simulink library "pmm"  (R2021b)
settings: Solver=VariableStepAuto  StartTime=0.0  StopTime=10.0  RelTol=1e-3
undefined symbols (not defined in the file or in its folder): APMM_CoolgFanActCurr_X_pct, APMM_EWP1Curr_X_c, APMM_EWP3Curr_X_c, APMM_LVBattChktime_X_enum, APMM_LVBattChrgtime_X_enum, APMM_LVChrgLv_X_mV, ENUM_ANTITHEFT_ALARM, ENUM_ANTITHEFT_ARM, ENUM_ANTITHEFT_DISARM, ENUM_ANTITHEFT_WAIT, ENUM_CHRGPLUGSTA_NONE, ENUM_CRASHSTATE_NOCRASH, ENUM_DCDCFAULTSTA_ANYFAULTLV1, ENUM_DCDCFAULTSTA_ANYFAULTLV2, ENUM_DRIVETRAIN_AWD, ENUM_DRIVETRAIN_FWD, ENUM_DRIVETRAIN_RWD, ENUM_GEARACTUALPOSN_D, ENUM_GEARACTUALPOSN_N, ENUM_GEARACTUALPOSN_R, ENUM_HVBATTREADYPRE_READY, ENUM_OTACHKSTA_NOREQUEST, ENUM_OTACHKSTA_NOTIMEOUT, ENUM_OTACHKSTA_TIMEOUT, ENUM_PDKEYRAWLULOCK_INLOCK, ENUM_PDKEYRAWLULOCK_INUNLOCK, ENUM_PDKEYRAWPS_INPS, ENUM_PDKEYSTA_LOCK, ENUM_PDKEYSTA_PS, ENUM_PDKEYSTA_UNAVALIABLE, ENUM_PDKEYSTA_UNLOCK, ENUM_POWERSTA_OFF, ENUM_POWERSTA_OFFC, ENUM_POWERSTA_STANDBY, ENUM_PWRREQOTA_REQPOWEROFF, ENUM_PWRREQOTA_REQPOWERSTDBY, ENUM_PWRSTASW_READY, FALSE, KPMM_AllDoorClosedHoldTime_s, KPMM_APSAllowThd_pct, KPMM_BattDownFailtime_s, KPMM_BattUpFailtime_s, KPMM_BattUpResetRty_cnt, KPMM_BattUpResetSW_flg, KPMM_BattUpResetTO_s, KPMM_BattUpRstDlyTO_s, KPMM_BrakeSWHoldTime_s, KPMM_ChrgPlugHoldTime_s, KPMM_DCDCDisableFailtime_s, KPMM_DCDCEnableFailtime_s, KPMM_DCDCVSET_V, KPMM_DCDCVSETLVChrg_V, KPMM_DoorSWHoldTime_s, KPMM_DriverSafetyChkFailtime_s, KPMM_DrivetrainSelect_enum_ovrdflg, KPMM_DrivetrainSelect_enum_ovrdval, KPMM_FDADC12VDetAccu_s, KPMM_FDADC12VDetAccuIntval_s, KPMM_FirstLVCheckHoldT_s, KPMM_FrMCUDischrgVolt_V ... (+54)
libraries: simulink x28, hcu_lib x13
(part 1 of 5)
settings Model: Creator=13615  LastModifiedBy=FVT23010
settings SolverCC: AlgebraicLoopSolver=TrustRegion
settings DataIOCC: SaveFormat=Array  SignalLoggingSaveFormat=ModelDataLogs  ReturnWorkspaceOutputs=off
settings OptimizationCC: BlockReduction=off  BooleanDataType=off
settings DebuggingCC: SaveWithParameterizedLinksMsg=none  UnderspecifiedInitializationDetection=Classic  MergeDetectMultiDrivingBlocksExec=none  SignalResolutionControl=TryResolveAllWithWarning  SFMachineParentedDataDiag=warning  ArithmeticOperatorsInVariantConditions=warning
settings HardwareCC: TargetUnknown=on
settings ModelReferenceCC: PropagateSignalLabelsOutOfModel=off
settings SFSimCC: SimUseLocalCustomCode=off  CustomCodeUndefinedFunction=UseInterfaceOnly
settings RTWCC: RTWUseLocalCustomCode=off
settings ConfigComp: CovMetricSettings=dw  CovSaveCumulativeToWorkspaceVar=on  CovSaveSingleToWorkspaceVar=on

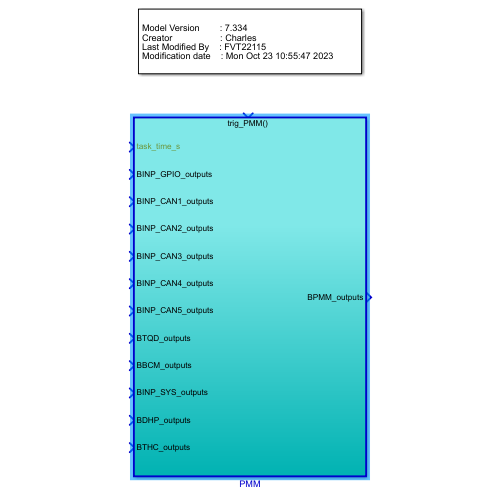
[thumbnail: Simulink's stored preview of the top-level diagram]
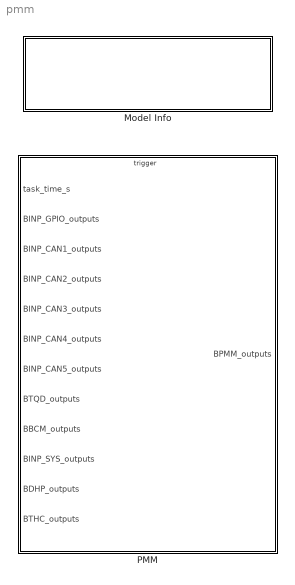
== system pmm ==
  Model Info : Subsystem  LoadFcn=slcm LoadBlock;  InitFcn=slcm('UpdateAllCMBlocksInThisModelInit')  mask(CMBlock){InitialSaveTempField=, InitialBlockCM=None, BlockCM=None, Frame=on, SaveTempField=, DisplayStringWithTags=|, MaskDisplayString=Model Version        : 7.543\nCreator                   : Charles\nLast Modified By    : FVT23010\nModification date    : Mon Jun 24 15:30:34 2024, HorizontalTextAlignment=Left, LeftAlignmentValue=0.02, SourceBlockDiagram=pmm, TagMaxNumber=20, CMTag1=, CMTag2=, CMTag3=, CMTag4=, CMTag5=, CMTag6=, CMTag7=, CMTag8=, CMTag9=, CMTag10=, CMTag11=, CMTag12=, CMTag13=, CMTag14=, CMTag15=, CMTag16=, CMTag17=, CMTag18=, CMTag19=, CMTag20=}
      mask DisplayStringWithTags=|
      | Model Version        : %<ModelVersion>
      | Creator                   : Charles
      | Last Modified By    : %<LastModifiedBy>
      | Modification date    : %<LastModificationDate>
      mask help: This block allows revision control information to be displayed within the model.
      settings: CopyFcn=slcm CopyBlock;  DeleteFcn=slcm Cancel;  PostSaveFcn=slcm('UpdateAllCMBlocksInThisModel')  NameChangeFcn=slcm Rename;  OpenFcn=slcm
      mask Display: text(str2num(LeftAlignmentValue), 0.5, MaskDisplayString, 'HorizontalAlignment', HorizontalTextAlignment)
  PMM : Subsystem  TreatAsAtomicUnit=on
      settings: RTWSystemCode=Nonreusable function  RTWFcnNameOpts=Use subsystem name  RTWFileNameOpts=Use subsystem name

== system pmm/Model Info ==
  EmptySubsystem : Subsystem

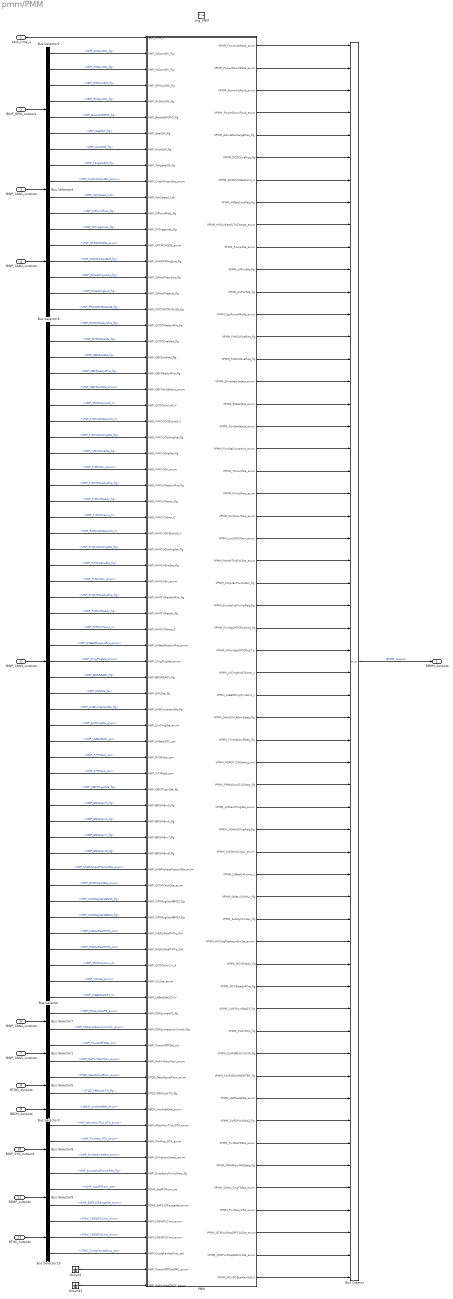
== system pmm/PMM ==
  task_time_s : Inport
  BINP_GPIO_outputs : Inport  Port=2  OutDataTypeStr=Bus: BINP_GPIO_outputs
  BINP_CAN1_outputs : Inport  Port=3  OutDataTypeStr=Bus: BINP_CAN1_outputs
  BINP_CAN2_outputs : Inport  Port=4  OutDataTypeStr=Bus: BINP_CAN2_outputs
  BINP_CAN3_outputs : Inport  Port=5  OutDataTypeStr=Bus: BINP_CAN3_outputs
  BINP_CAN4_outputs : Inport  Port=6  OutDataTypeStr=Bus: BINP_CAN4_outputs
  BINP_CAN5_outputs : Inport  Port=7  OutDataTypeStr=Bus: BINP_CAN5_outputs
  BTQD_outputs : Inport  Port=8  OutDataTypeStr=Bus: BTQD_outputs
  BBCM_outputs : Inport  Port=9  OutDataTypeStr=Bus: BBCM_outputs
  BINP_SYS_outputs : Inport  Port=10  OutDataTypeStr=Bus: BINP_SYS_outputs
  BDHP_outputs : Inport  Port=11  OutDataTypeStr=Bus: BDHP_outputs
  BTHC_outputs : Inport  Port=12  OutDataTypeStr=Bus: BTHC_outputs
  trig_PMM : TriggerPort  TriggerType=function-call  VariantControl=(inherit)
  Bus Creator : BusCreator  Inputs=56  OutDataTypeStr=Bus: BPMM_outputs  NonVirtualBus=on
  Bus Selector : BusSelector  OutputSignals=VINP_DCDCReady4Pre_flg,VINP_DCDCEnaSta_flg,VINP_OBCEnaSta_flg,VINP_OBCReady4Pre_flg,VINP_OBCFaultSta_enum,VINP_DCDCAuxVolt_V,VINP_FrMCUDCBusVolt_V,VINP_FrMCUDischrgSta_flg,VINP_FrMCUEnaSta_flg,VINP_FrMCUErr_enum,VINP_FrMCUReady4Pre_flg,VINP_FrMCUReady_flg,VINP_FrMCUTemp_C,VINP_RrMCUDCBusVolt_V,VINP_RrMCUDischrgSta_flg,VINP_RrMCUEnaSta_flg,VINP_RrMCUErr_enum,VINP_RrMCUReady4Pre_flg,VINP_RrMCUReady_flg,VINP_RrMCUTemp_C,VINP_HVBattReady4Pre_enum,VINP_ChrgPlugSta_enum,VINP_BMSREADY_flg,VINP_HVILSta_flg,VINP_HVBContactorSta_flg,VINP_ExtChrgSta_enum,VINP_HVBattSOC_pct,VINP_RrTMSpd_rpm,VINP_FrTMSpd_rpm,VINP_OBCPluginSta_flg,VINP_BMSWarn5_flg,VINP_BMSWarn6_flg,VINP_BMSWarn7_flg,VINP_BMSWarn8_flg,VINP_HVBPreheatPrecoolSta_enum,VINP_DCDCFaultSta_enum,VINP_CANMsgValidBMS5_flg,VINP_CANMsgValidBMS3_flg,VINP_FrEDURealTMTq_Nm,VINP_RrEDURealTMTq_Nm,VINP_DCDCAuxCur_A,VINP_V2LSta_enum,VINP_LVBattDet12V_V
  Bus Selector1 : BusSelector  OutputSignals=VINP_PowerOffTSet_cnt,VINP_RePwrReqTbox_enum
  Bus Selector10 : BusSelector  OutputSignals=VTHC_FDEWP1Cmd_enum,VTHC_FDEWP3Cmd_enum,VTHC_CoolgFanActDuty_pct
  Bus Selector2 : BusSelector  OutputSignals=VINP_DrDoorSW_flg,VINP_PsDoorSW_flg,VINP_RRDoorSW_flg,VINP_RLDoorSW_flg,VINP_BrakeSWGPIO_flg,VINP_SeatSW_flg,VINP_HoodSW_flg,VINP_TailgateSW_flg
  Bus Selector3 : BusSelector  OutputSignals=VBCM_AntitheftSta_enum
  Bus Selector4 : BusSelector  OutputSignals=VINP_CrashOutputSts_enum,VINP_VehSpeed_kph
  Bus Selector5 : BusSelector  OutputSignals=VTQD_GearActualPosn_enum,VTQD_PBWLockTO_flg
  Bus Selector6 : BusSelector  OutputSignals=VINP_IVIPwroffreq_flg,VINP_IVITriggerreq_flg,VINP_OFFACMODE_enum,VINP_AVMOFFRecButt_flg,VINP_SchedChgwake_flg,VINP_SchedChgbutt_flg,VINP_PWCONTINUEUSE_flg
  Bus Selector7 : BusSelector  OutputSignals=VINP_PDKeyAreaPS_enum,VINP_PDKeyAreaLockUnlock_enum
  Bus Selector8 : BusSelector  OutputSignals=VINP_AllowMovThd_OTA_enum,VINP_PwrReq_OTA_enum,VINP_DrivetrainSelect_enum,VINP_EvccAplusPwrUpReq_flg
  Bus Selector9 : BusSelector  OutputSignals=VDHP_ActAPSPosn_pct,VDHP_EAPS12RangeSta_enum
  Ground : Ground
  Ground3 : Ground
  PMM : Subsystem
  BPMM_outputs : Outport  OutDataTypeStr=Bus: BPMM_outputs  VectorParamsAs1DForOutWhenUnconnected=off
  wires:
  BINP_CAN3_outputs/1 -> Bus Selector/1
  Bus Creator/1 -> BPMM_outputs/1  "BPMM_outputs"
  task_time_s/1 -> PMM/1(task_time_s)
  BINP_GPIO_outputs/1 -> Bus Selector2/1
  BBCM_outputs/1 -> Bus Selector3/1
  BTQD_outputs/1 -> Bus Selector5/1
  Bus Selector2/4 -> PMM/5(VINP_RLDoorSW_flg)  "<VINP_RLDoorSW_flg>"
  Bus Selector2/5 -> PMM/6(VINP_BrakeSWGPIO_flg)  "<VINP_BrakeSWGPIO_flg>"
  Bus Selector2/3 -> PMM/4(VINP_RRDoorSW_flg)  "<VINP_RRDoorSW_flg>"
  Bus Selector2/2 -> PMM/3(VINP_PsDoorSW_flg)  "<VINP_PsDoorSW_flg>"
  Bus Selector2/1 -> PMM/2(VINP_DrDoorSW_flg)  "<VINP_DrDoorSW_flg>"
  Bus Selector/1 -> PMM/19(VINP_DCDCReady4Pre_flg)  "<VINP_DCDCReady4Pre_flg>"
  Bus Selector/2 -> PMM/20(VINP_DCDCEnabled_flg)  "<VINP_DCDCEnaSta_flg>"
  Bus Selector/3 -> PMM/21(VINP_OBCEnabled_flg)  "<VINP_OBCEnaSta_flg>"
  Bus Selector/4 -> PMM/22(VINP_OBCReady4Pre_flg)  "<VINP_OBCReady4Pre_flg>"
  Bus Selector/5 -> PMM/23(VINP_OBCFaultStatus_enum)  "<VINP_OBCFaultSta_enum>"
  Bus Selector/6 -> PMM/24(VINP_DCDCAuxVolt_V)  "<VINP_DCDCAuxVolt_V>"
  Bus Selector/7 -> PMM/25(VINP_FrMCUDCBusVolt_V)  "<VINP_FrMCUDCBusVolt_V>"
  Bus Selector/8 -> PMM/26(VINP_FrMCUDischrgSta_flg)  "<VINP_FrMCUDischrgSta_flg>"
  Bus Selector/9 -> PMM/27(VINP_FrMCUEnaSta_flg)  "<VINP_FrMCUEnaSta_flg>"
  Bus Selector/10 -> PMM/28(VINP_FrMCUErr_enum)  "<VINP_FrMCUErr_enum>"
  Bus Selector/11 -> PMM/29(VINP_FrMCUReady4Pre_flg)  "<VINP_FrMCUReady4Pre_flg>"
  Bus Selector/12 -> PMM/30(VINP_FrMCUReady_flg)  "<VINP_FrMCUReady_flg>"
  Bus Selector/13 -> PMM/31(VINP_FrMCUTemp_C)  "<VINP_FrMCUTemp_C>"
  Bus Selector/14 -> PMM/32(VINP_RrMCUDCBusVolt_V)  "<VINP_RrMCUDCBusVolt_V>"
  Bus Selector/15 -> PMM/33(VINP_RrMCUDischrgSta_flg)  "<VINP_RrMCUDischrgSta_flg>"
  Bus Selector/16 -> PMM/34(VINP_RrMCUEnaSta_flg)  "<VINP_RrMCUEnaSta_flg>"
  Bus Selector/17 -> PMM/35(VINP_RrMCUErr_enum)  "<VINP_RrMCUErr_enum>"
  Bus Selector/18 -> PMM/36(VINP_RrMCUReady4Pre_flg)  "<VINP_RrMCUReady4Pre_flg>"
  Bus Selector/19 -> PMM/37(VINP_RrMCUReady_flg)  "<VINP_RrMCUReady_flg>"
  Bus Selector/20 -> PMM/38(VINP_RrMCUTemp_C)  "<VINP_RrMCUTemp_C>"
  Bus Selector/21 -> PMM/39(VINP_HVBattReady4Pre_enum)  "<VINP_HVBattReady4Pre_enum>"
  Bus Selector/22 -> PMM/40(VINP_ChrgPlugSta_enum)  "<VINP_ChrgPlugSta_enum>"
  Bus Selector/23 -> PMM/41(VINP_BMSREADY_flg)  "<VINP_BMSREADY_flg>"
  Bus Selector/24 -> PMM/42(VINP_HVILSta_flg)  "<VINP_HVILSta_flg>"
  Bus Selector/26 -> PMM/44(VINP_ExtChrgSta_enum)  "<VINP_ExtChrgSta_enum>"
  BINP_CAN1_outputs/1 -> Bus Selector4/1
  Bus Selector4/1 -> PMM/10(VINP_CrashOutputSts_enum)  "<VINP_CrashOutputSts_enum>"
  Bus Selector2/6 -> PMM/7(VINP_SeatSW_flg)  "<VINP_SeatSW_flg>"
  Bus Selector/27 -> PMM/45(VINP_HVBattSOC_pct)  "<VINP_HVBattSOC_pct>"
  Bus Selector/25 -> PMM/43(VINP_HVBContactorSta_flg)  "<VINP_HVBContactorSta_flg>"
  BINP_CAN2_outputs/1 -> Bus Selector6/1
  Bus Selector6/1 -> PMM/12(VINP_IVIPwroffreq_flg)  "<VINP_IVIPwroffreq_flg>"
  Bus Selector6/2 -> PMM/13(VINP_IVITriggerreq_flg)  "<VINP_IVITriggerreq_flg>"
  Bus Selector7/1 -> PMM/62(VINP_PDKeyAreaPS_flg)  "<VINP_PDKeyAreaPS_enum>"
  Bus Selector7/2 -> PMM/63(VINP_PDKeyAreaLockUnlock_flg)  "<VINP_PDKeyAreaLockUnlock_enum>"
  BINP_CAN4_outputs/1 -> Bus Selector7/1
  Bus Selector/28 -> PMM/46(VINP_RrTMSpd_rpm)  "<VINP_RrTMSpd_rpm>"
  Bus Selector4/2 -> PMM/11(VINP_VehSpeed_kph)  "<VINP_VehSpeed_kph>"
  Bus Selector/29 -> PMM/47(VINP_FrTMSpd_rpm)  "<VINP_FrTMSpd_rpm>"
  Bus Selector6/3 -> PMM/14(VINP_OFFACMODE_enum)  "<VINP_OFFACMODE_enum>"
  Bus Selector/30 -> PMM/48(VINP_OBCPluginSta_flg)  "<VINP_OBCPluginSta_flg>"
  Bus Selector/31 -> PMM/49(VINP_BMSWarn5_flg)  "<VINP_BMSWarn5_flg>"
  Bus Selector/32 -> PMM/50(VINP_BMSWarn6_flg)  "<VINP_BMSWarn6_flg>"
  Bus Selector/33 -> PMM/51(VINP_BMSWarn7_flg)  "<VINP_BMSWarn7_flg>"
  Bus Selector/34 -> PMM/52(VINP_BMSWarn8_flg)  "<VINP_BMSWarn8_flg>"
  BINP_CAN5_outputs/1 -> Bus Selector1/1
  Bus Selector/35 -> PMM/53(VINP_HVBPreheatPrecoolSta_enum)  "<VINP_HVBPreheatPrecoolSta_enum>"
  Bus Selector6/4 -> PMM/15(VINP_AVMOFFRecButt_flg)  "<VINP_AVMOFFRecButt_flg>"
  Bus Selector6/5 -> PMM/16(VINP_SchedChgwake_flg)  "<VINP_SchedChgwake_flg>"
  Bus Selector2/7 -> PMM/8(VINP_HoodSW_flg)  "<VINP_HoodSW_flg>"
  Bus Selector2/8 -> PMM/9(VINP_TailgateSW_flg)  "<VINP_TailgateSW_flg>"
  Bus Selector6/6 -> PMM/17(VINP_SchedChgbutt_flg)  "<VINP_SchedChgbutt_flg>"
  Bus Selector/38 -> PMM/56(VINP_CANMsgValidBMS3_flg)  "<VINP_CANMsgValidBMS3_flg>"
  BINP_SYS_outputs/1 -> Bus Selector8/1
  Bus Selector8/1 -> PMM/69(VINP_AllowMovThd_OTA_enum)  "<VINP_AllowMovThd_OTA_enum>"
  Bus Selector8/2 -> PMM/70(VINP_PwrReq_OTA_enum)  "<VINP_PwrReq_OTA_enum>"
  Bus Selector3/1 -> PMM/68(VBCM_AntitheftSta_enum)  "<VBCM_AntitheftSta_enum>"
  Bus Selector5/1 -> PMM/66(VTQD_GearActualPosn_enum)  "<VTQD_GearActualPosn_enum>"
  Bus Selector5/2 -> PMM/67(VTQD_PBWLockTO_flg)  "<VTQD_PBWLockTO_flg>"
  Ground3/1 -> PMM/79(VINP_RePwrReqDKCT_enum)
  Ground/1 -> PMM/78(VINP_PowerOffTSetDKC_enum)
  Bus Selector1/1 -> PMM/64(VINP_PowerOffTSet_cnt)  "<VINP_PowerOffTSet_cnt>"
  Bus Selector1/2 -> PMM/65(VINP_RePwrReqTbox_enum)  "<VINP_RePwrReqTbox_enum>"
  Bus Selector8/3 -> PMM/71(VINP_DrivetrainSelect_enum)  "<VINP_DrivetrainSelect_enum>"
  Bus Selector8/4 -> PMM/72(VINP_EvccAplusPwrUpReq_flg)  "<VINP_EvccAplusPwrUpReq_flg>"
  BDHP_outputs/1 -> Bus Selector9/1
  Bus Selector9/1 -> PMM/73(VDHP_ActAPSPosn_pct)  "<VDHP_ActAPSPosn_pct>"
  Bus Selector/36 -> PMM/54(VINP_DCDCFaultSta_enum)  "<VINP_DCDCFaultSta_enum>"
  Bus Selector/39 -> PMM/57(VINP_FrEDURealTMTq_Nm)  "<VINP_FrEDURealTMTq_Nm>"
  Bus Selector/40 -> PMM/58(VINP_RrEDURealTMTq_Nm)  "<VINP_RrEDURealTMTq_Nm>"
  Bus Selector/41 -> PMM/59(VINP_DCDCAuxCur_A)  "<VINP_DCDCAuxCur_A>"
  BTHC_outputs/1 -> Bus Selector10/1
  Bus Selector10/1 -> PMM/75(VINP_FDEWP1Cmd_enum)  "<VTHC_FDEWP1Cmd_enum>"
  Bus Selector10/2 -> PMM/76(VINP_FDEWP3Cmd_enum)  "<VTHC_FDEWP3Cmd_enum>"
  Bus Selector10/3 -> PMM/77(VINP_CoolgFanActDuty_pct)  "<VTHC_CoolgFanActDuty_pct>"
  Bus Selector6/7 -> PMM/18(VINP_PWCONTINUEUSE_flg)  "<VINP_PWCONTINUEUSE_flg>"
  PMM/1(VPMM_PowerUpState_enum) -> Bus Creator/1
  PMM/2(VPMM_PowerDownState_enum) -> Bus Creator/2
  PMM/3(VPMM_PowerUpFault_enum) -> Bus Creator/3
  PMM/4(VPMM_PowerDownFault_enum) -> Bus Creator/4
  PMM/5(VPMM_ActiveDischargeReq_flg) -> Bus Creator/5
  PMM/6(VPMM_DCDCEnaReq_flg) -> Bus Creator/6
  PMM/7(VPMM_DCDCVoltSetpoint_V) -> Bus Creator/7
  PMM/8(VPMM_HVBatCnctReq_flg) -> Bus Creator/8
  PMM/9(VPMM_HVSysReadyToCharge_enum) -> Bus Creator/9
  PMM/10(VPMM_PowerSta_enum) -> Bus Creator/10
  PMM/11(VPMM_LVPwrSta_flg) -> Bus Creator/11
  PMM/12(VPMM_HVPwrSta_flg) -> Bus Creator/12
  PMM/13(VPMM_SysPowerMode_enum) -> Bus Creator/13
  PMM/14(VPMM_FrMCUEnaReq_flg) -> Bus Creator/14
  PMM/15(VPMM_RrMCUEnaReq_flg) -> Bus Creator/15
  PMM/16(VPMM_DrivetrainSelect_enum) -> Bus Creator/16
  PMM/17(VPMM_DrSeatSta_enum) -> Bus Creator/17
  PMM/18(VPMM_PwrStaSelect_enum) -> Bus Creator/18
  PMM/19(VPMM_PwrStaConstraint_enum) -> Bus Creator/19
  PMM/20(VPMM_TCountSta_enum) -> Bus Creator/20
  PMM/21(VPMM_PwrUpReq_enum) -> Bus Creator/21
  PMM/22(VPMM_PwrDownReq_enum) -> Bus Creator/22
  PMM/23(VPMM_LowSOCWarn_enum) -> Bus Creator/23
  PMM/24(VPMM_ReVehThdChkSta_enum) -> Bus Creator/24
  PMM/25(VPMM_LVSysErrPwrOutErr_flg) -> Bus Creator/25
  PMM/26(VPMM_EvccAplusPwrUpReq_flg) -> Bus Creator/26
  PMM/27(VPMM_PwrStaONTOPopReq_flg) -> Bus Creator/27
  PMM/28(VPMM_IVIPwrStaONTOPopT_s) -> Bus Creator/28
  PMM/29(VPMM_LVChrgHoldTtimer_s) -> Bus Creator/29
  PMM/30(VPMM_LVBattChrgTimeCnt_s) -> Bus Creator/30
  PMM/31(VPMM_SilentChkAllowSleep_flg) -> Bus Creator/31
  PMM/32(VPMM_TimerAllowSleep_flg) -> Bus Creator/32
  PMM/33(VPMM_FDADC12VDetAvg_mV) -> Bus Creator/33
  PMM/34(VPMM_PMMAllowECUSleep_flg) -> Bus Creator/34
  PMM/35(VPMM_LVSilentChrgSta_enum) -> Bus Creator/35
  PMM/36(VPMM_LVSilentChrgReq_flg) -> Bus Creator/36
  PMM/37(VPMM_LVSilentChrgLv_enum) -> Bus Creator/37
  PMM/38(VPMM_LVBattChktime_s) -> Bus Creator/38
  Bus Selector/37 -> PMM/55(VINP_CANMsgValidBMS2_flg)  "<VINP_CANMsgValidBMS5_flg>"
  PMM/39(VPMM_SafetyChkMLv_flg) -> Bus Creator/39
  PMM/40(VPMM_SafetyChkHLv_flg) -> Bus Creator/40
  PMM/41(VPMM_HVChrgPreActionErrSta_enum) -> Bus Creator/41
  PMM/42(VPMM_MCUReady_flg) -> Bus Creator/42
  PMM/43(VPMM_MCUReady4Pre_flg) -> Bus Creator/43
  PMM/44(VPMM_CtrlFrPwrStbA1P_flg) -> Bus Creator/44
  PMM/45(VPMM_CtrlFrRC1_flg) -> Bus Creator/45
  PMM/46(VPMM_CtrlFrBMSCCUCIR_flg) -> Bus Creator/46
  PMM/47(VPMM_CtrlFrEDUINVERTER_flg) -> Bus Creator/47
  PMM/48(VPMM_HWResetSta_enum) -> Bus Creator/48
  PMM/49(VPMM_CtrlDrPwrStbA2_flg) -> Bus Creator/49
  Bus Selector9/2 -> PMM/74(VDHP_EAPS12RangeSta_enum)  "<VDHP_EAPS12RangeSta_enum>"
  PMM/50(VPMM_PwrStaTOSta_enum) -> Bus Creator/50
  Bus Selector/42 -> PMM/60(VINP_V2LSta_enum)  "<VINP_V2LSta_enum>"
  PMM/51(VPMM_PMMAllowNMSleep_flg) -> Bus Creator/51
  Bus Selector/43 -> PMM/61(VINP_LVBattDet12V_V)  "<VINP_LVBattDet12V_V>"
  PMM/52(VPMM_Sched_ChgTOSta_enum) -> Bus Creator/52
  PMM/53(VPMM_PwrReq_OTA_enum) -> Bus Creator/53
  PMM/54(VPMM_OTAPwrReqOFFChkSta_enum) -> Bus Creator/54
  PMM/55(VPMM_OTAPwrReqStdChkSta_enum) -> Bus Creator/55
  PMM/56(VPMM_MCUDCBusMaxVolt_V) -> Bus Creator/56

== system pmm/Model Info/EmptySubsystem ==
